simulink model "abfilter"  (Simulink 8.0)
settings: Solver=FixedStepDiscrete  StartTime=0.0  StopTime=10  FixedStep=T  RelTol=1e-3
InitFcn:
  | init
values from neighbouring files (symbols this model uses):
  a = 0.8    [init.m]
  b = 0.2    [init.m]
  T = 0.1    [init.m]
undefined symbols (not defined in the file or in its folder): DiscIntNeverNeededParam
libraries: commchan3 x1, simulink x1
settings Model: Creator=m.rodkin  LastModifiedBy=mishuk
settings DataIOCC: SignalLoggingSaveFormat=ModelDataLogs
settings DebuggingCC: FcnCallInpInsideContextMsg=UseLocalSettings  StrictBusMsg=Warning
settings SFSimCC: SimParseCustomCode=off
settings GRTTargetCC: CombineOutputUpdateFcns=off  GRTInterface=on

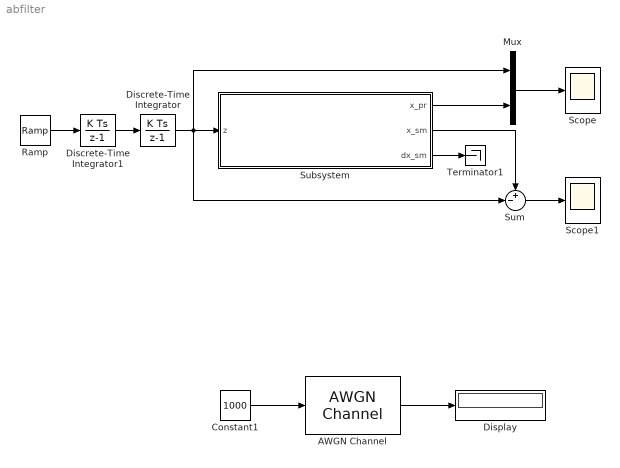
== system abfilter ==
  AWGN Channel : commchan3/AWGN Channel  InputProcessing=Inherited (this choice will be removed - see release notes)  seed=67  noiseMode=Variance from mask  EbNodB=10  EsNodB=10  SNRdB=10  bitsPerSym=1  Ps=1  Tsym=1  variance=0.1
  Constant1 : Constant  Value=1000
  Discrete-Time Integrator : DiscreteIntegrator  SampleTime=T  ICPrevOutput=DiscIntNeverNeededParam  ICPrevScaledInput=DiscIntNeverNeededParam
  Discrete-Time Integrator1 : DiscreteIntegrator  SampleTime=T  ICPrevOutput=DiscIntNeverNeededParam  ICPrevScaledInput=DiscIntNeverNeededParam
  Display : Display
  Mux : Mux  Inputs=2
  Ramp : simulink/Sources/Ramp  slope=1  start=0  X0=0
  Scope : Scope
  Scope1 : Scope
  Subsystem : Subsystem  mask{a=a, b=b}
      mask prompts: a "Alpha"; b "Beta"
      mask Display:
      | fprintf('AB\n filter')
      | port_label('input', 1, 'z')
      | port_label('output', 1, 'x_pr')
      | port_label('output', 2, 'x_sm')
      | port_label('output', 3, 'dx_sm')
  Sum : Sum  Inputs=+-|
  Terminator1 : Terminator
  wires:
  Subsystem/3(dx_sm) -> Terminator1/1
  AWGN Channel/1 -> Display/1
  Discrete-Time Integrator/1 -> Mux/1, Sum/2, Subsystem/1(z)
  Subsystem/2(x_sm) -> Sum/1
  Mux/1 -> Scope/1
  Subsystem/1(x_pr) -> Mux/2
  Sum/1 -> Scope1/1
  Constant1/1 -> AWGN Channel/1
  Discrete-Time Integrator1/1 -> Discrete-Time Integrator/1
  Ramp/1 -> Discrete-Time Integrator1/1

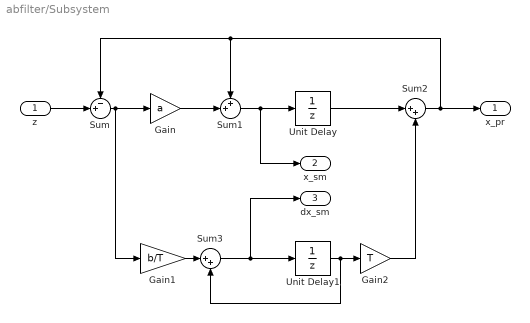
== system abfilter/Subsystem ==
  z : Inport
  Gain : Gain  Gain=a
  Gain1 : Gain  Gain=b/T
  Gain2 : Gain  Gain=T
  Sum : Sum  Inputs=-+|
  Sum1 : Sum  Inputs=++|
  Sum2 : Sum  Inputs=|++
  Sum3 : Sum  Inputs=|++
  Unit Delay : UnitDelay  SampleTime=-1
  Unit Delay1 : UnitDelay  SampleTime=-1
  x_pr : Outport
  x_sm : Outport  Port=2
  dx_sm : Outport  Port=3
  wires:
  z/1 -> Sum/2
  Sum/1 -> Gain/1, Gain1/1
  Gain/1 -> Sum1/2
  Sum1/1 -> Unit Delay/1, x_sm/1
  Unit Delay/1 -> Sum2/1
  Sum2/1 -> x_pr/1, Sum/1, Sum1/1
  Gain1/1 -> Sum3/1
  Sum3/1 -> Unit Delay1/1, dx_sm/1
  Unit Delay1/1 -> Gain2/1, Sum3/2
  Gain2/1 -> Sum2/2
